simulink model "first_simulink_model"  (R2020a)
settings: Solver=VariableStepAuto  StartTime=0.0  StopTime=10  RelTol=1e-3
libraries: simulink x2
settings Model: Creator=joshi  LastModifiedBy=joshi

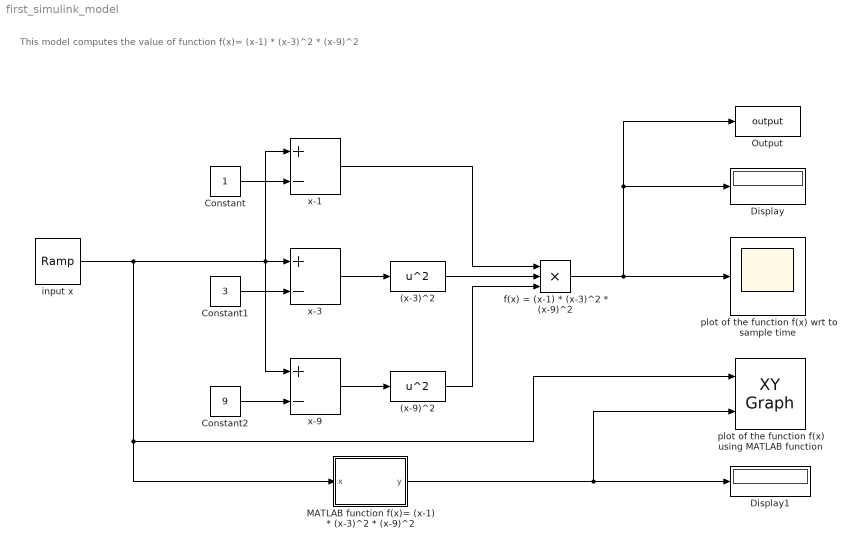
== system first_simulink_model ==
  note: This model computes the value of function
      | f(x)= (x-1) * (x-3)^2 * (x-9)^2
  " f(x) = (x-1) * (x-3)^2 * (x-9)^2" : Product  Inputs=3
  (x-3)^2 : Math  Operator=square  SaturateOnIntegerOverflow=on
  (x-9)^2 : Math  Operator=square  SaturateOnIntegerOverflow=on
  Constant : Constant
  Constant1 : Constant  Value=3
  Constant2 : Constant  Value=9
  Display : Display
  Display1 : Display
  "MATLAB function f(x)= (x-1) * (x-3)^2 * (x-9)^2 " : MATLAB Function  TreatAsAtomicUnit=on
  "Output " : ToWorkspace  VariableName=output  SaveFormat=Timeseries  SampleTime=-1
  input x : simulink/Sources/Ramp  slope=1  start=0  InitialOutput=0
  plot of the function f(x) using MATLAB function : simulink/Sinks/XY Graph  xmin=0  xmax=10  ymin=-900  ymax=500  st=-1
  plot of the function f(x) wrt to sample time : Scope
  x-1 : Sum  Inputs=+-
  x-3 : Sum  Inputs=+-
  x-9 : Sum  Inputs=+-
  wires:
  Constant/1 -> x-1/2
  input x/1 -> plot of the function f(x) using MATLAB function/1, "MATLAB function f(x)= (x-1) * (x-3)^2 * (x-9)^2 "/1(x), x-3/1, x-1/1, x-9/1
  Constant1/1 -> x-3/2
  Constant2/1 -> x-9/2
  x-3/1 -> (x-3)^2/1
  x-9/1 -> (x-9)^2/1
  x-1/1 -> " f(x) = (x-1) * (x-3)^2 * (x-9)^2"/1
  (x-3)^2/1 -> " f(x) = (x-1) * (x-3)^2 * (x-9)^2"/2
  (x-9)^2/1 -> " f(x) = (x-1) * (x-3)^2 * (x-9)^2"/3
  " f(x) = (x-1) * (x-3)^2 * (x-9)^2"/1 -> "Output "/1, Display/1, plot of the function f(x) wrt to sample time/1
  "MATLAB function f(x)= (x-1) * (x-3)^2 * (x-9)^2 "/1(y) -> plot of the function f(x) using MATLAB function/2, Display1/1

== matlab function first_simulink_model/MATLAB function f(x)= (x-1) * (x-3)^2 * (x-9)^2  ==
  data: x input; y output
function y = fcn(x)

 
 y = (x-1) * (x-3)^2 * (x-9)^2;
end
